simulink model "svpwm_twolevel"  (R2020a)
settings: Solver=ode45  StartTime=0.0  StopTime=0.05  RelTol=1e-3  EnableMultiTasking=on
libraries: powerlib x15, simulink x1
settings Model: Creator=Lenovo  LastModifiedBy=DELL
settings DataIOCC: LimitDataPoints=on  SaveFormat=Array  ReturnWorkspaceOutputs=off
settings OptimizationCC: LifeSpan=inf
settings DebuggingCC: SFUnexpectedBacktrackingDiag=warning  SFNoUnconditionalDefaultTransitionDiag=warning  SFExecutionAtInitializationDiag=none  ArithmeticOperatorsInVariantConditions=warning
settings HardwareCC: ProdBitPerPointer=32  ProdBitPerSizeT=32  ProdBitPerPtrDiffT=32  ProdLargestAtomicFloat=None  ProdIntDivRoundTo=Undefined  ProdEndianess=Unspecified  ProdWordSize=32  ProdHWDeviceType=32-bit Generic
settings ModelReferenceCC: PropagateSignalLabelsOutOfModel=off
settings SFSimCC: SimUseLocalCustomCode=off  CustomCodeUndefinedFunction=UseInterfaceOnly
settings RTWCC: RTWUseLocalCustomCode=off
settings CodeAppCC: StateflowObjectComments=on
settings GRTTargetCC: TargetLangStandard=C89/C90 (ANSI)
settings ConfigComp: CovMetricSettings=dw  CovHtmlReporting=on  CovSaveCumulativeToWorkspaceVar=on  CovSaveSingleToWorkspaceVar=on  CovExternalEMLEnable=off
settings SimscapeCC: SimscapeNormalizeSystem=off

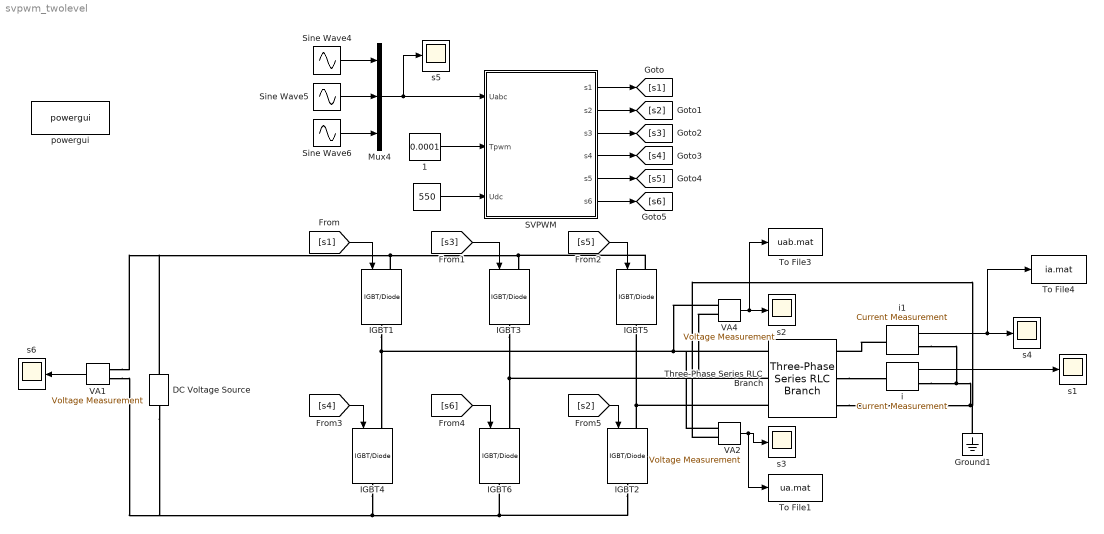
== system svpwm_twolevel ==
  " " : Constant  Value=550
  " 1" : Constant  Value=0.0001
  DC Voltage Source : powerlib/Electrical Sources/DC Voltage Source  Amplitude=550  Measurements=Voltage
  Ground1 : powerlib/Elements/Ground  LConnTagsString=a
  IGBT{1..6} (6 alike) : powerlib/Power Electronics/IGBT//Diode  Ron=1e-3  Rs=1e5  Cs=inf  Measurements=off
  Mux4 : Mux  Inputs=3
  SVPWM : Subsystem
  Sine Wave4 : Sin  Amplitude=200  Frequency=100*pi  SampleTime=0
  Sine Wave5 : Sin  Amplitude=200  Frequency=100*pi  Phase=-2*pi/3  SampleTime=0
  Sine Wave6 : Sin  Amplitude=200  Frequency=100*pi  Phase=-4*pi/3  SampleTime=0
  Three-Phase Series RLC Branch : powerlib/Elements/Three-Phase Series RLC Branch  LConnTagsString=A|B|C  RConnTagsString=A|B|C  BranchType=RL  Resistance=10  Inductance=1e-2  Capacitance=1e-6  Measurements=None
  To File1 : ToFile  Filename=ua.mat
  To File3 : ToFile  Filename=uab.mat
  To File4 : ToFile  Filename=ia.mat
  VA1 : powerlib/Measurements/Voltage Measurement  PhasorSimulation=off  OutputType=Complex  PSBequivalent=0
  VA2 : powerlib/Measurements/Voltage Measurement  PhasorSimulation=off  OutputType=Complex  PSBequivalent=0
  VA4 : powerlib/Measurements/Voltage Measurement  PhasorSimulation=off  OutputType=Complex  PSBequivalent=0
  i : powerlib/Measurements/Current Measurement  PhasorSimulation=off  OutputType=Complex  PSBequivalent=0
  i1 : powerlib/Measurements/Current Measurement  PhasorSimulation=off  OutputType=Complex  PSBequivalent=0
  powergui : powerlib/powergui  Priority=1  SimulationMode=Continuous  SampleTime=1e-6  frequency=60  Iterations=50  frequencyindice=0  Pbase=100e6  ErrMax=1e-4  UnitsV=V  UnitsW=MW  buscounter=0  FunctionMessages=off  echomessages=off  EnableUseOfTLC=off  CurrentSourceSwitches=off  DisableSnubberDevices=off  DisableRonSwitches=off  DisableVfSwitches=off  DisplayEquations=off  AutomaticDiscreteSolvers=off  SolverType=Tustin/Backward Euler (TBE)  Interpol=off  ExternalGateDelay=off  methode=off  Ts=100  x0status=blocks  SPID=off  SwTol=0  HookPort=off  NonlinearTolerance=1e-4  nMaxIteration=100  ContinueOnMaxIteration=off  RestoreLinks=warning  ResistiveCurrentMeasurement=off  Frange=[0:2:500]  Ylog=off  Xlog=on  ShowGrid=off  save=off  variable=ZData  structure=aa3  ZoomFFT=off  StartTime=0.5  cycles=19  DisplayStyle=1  fundamental=50  FreqAxis=off  MaxFrequency=770  frequencyindicesteady=1  RmsSteady=1  display=off
  s{1..6} (6 alike) : Scope
  wires:
  Mux4/1 -> s5/1, SVPWM/1(Uabc)
  " "/1 -> SVPWM/3(Udc)
  " 1"/1 -> SVPWM/2(Tpwm)
  Sine Wave4/1 -> Mux4/1
  Sine Wave5/1 -> Mux4/2
  Sine Wave6/1 -> Mux4/3
  SVPWM/1(s1) -> [s1]
  SVPWM/2(s2) -> [s2]
  SVPWM/3(s3) -> [s3]
  SVPWM/4(s4) -> [s4]
  SVPWM/5(s5) -> [s5]
  SVPWM/6(s6) -> [s6]
  [s1] -> IGBT1/1
  [s3] -> IGBT3/1
  [s5] -> IGBT5/1
  [s4] -> IGBT4/1
  [s6] -> IGBT6/1
  [s2] -> IGBT2/1
  VA1/1 -> s6/1
  i/1 -> s1/1
  VA4/1 -> To File3/1, s2/1
  VA2/1 -> To File1/1, s3/1
  i1/1 -> To File4/1, s4/1
  connections:
  IGBT1/LConn1 -- DC Voltage Source/RConn1 -- VA1/LConn1 -- IGBT5/LConn1 -- IGBT3/LConn1
  IGBT4/RConn1 -- DC Voltage Source/LConn1 -- VA1/LConn2 -- IGBT6/RConn1 -- IGBT2/RConn1
  IGBT1/RConn1 -- VA2/LConn1 -- Three-Phase Series RLC Branch/LConn1 -- VA4/LConn1 -- IGBT4/LConn1
  IGBT2/LConn1 -- IGBT5/RConn1 -- Three-Phase Series RLC Branch/LConn3
  IGBT3/RConn1 -- VA4/LConn2 -- Three-Phase Series RLC Branch/LConn2 -- IGBT6/LConn1
  Three-Phase Series RLC Branch/RConn2 -- i/LConn1
  i/RConn1 -- i1/RConn1 -- Ground1/LConn1 -- VA2/LConn2 -- Three-Phase Series RLC Branch/RConn3
  i1/LConn1 -- Three-Phase Series RLC Branch/RConn1

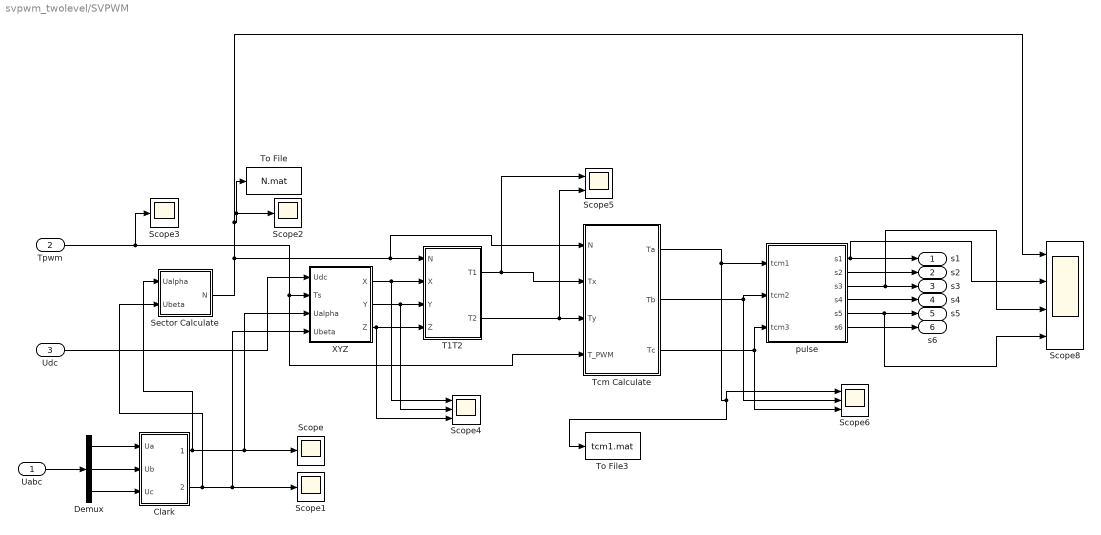
== system svpwm_twolevel/SVPWM ==
  Uabc : Inport
  Tpwm : Inport  Port=2
  Udc : Inport  Port=3
  Clark : Subsystem
  Demux : Demux  Outputs=3
  Scope{,1..3} (4 alike) : Scope
  Scope4 : Scope  NumInputPorts=3
  Scope5 : Scope  NumInputPorts=2
  Scope6 : Scope  NumInputPorts=3
  Scope8 : Scope  NumInputPorts=4
  Sector Calculate : Subsystem
  T1T2 : Subsystem
  Tcm Calculate : Subsystem
  To File : ToFile  Filename=N.mat
  To File3 : ToFile  Filename=tcm1.mat
  XYZ : Subsystem
  pulse : Subsystem
  s1 : Outport
  s2 : Outport  Port=2
  s3 : Outport  Port=3
  s4 : Outport  Port=4
  s5 : Outport  Port=5
  s6 : Outport  Port=6
  wires:
  XYZ/1(X) -> Scope4/1, T1T2/2(X)
  XYZ/2(Y) -> Scope4/2, T1T2/3(Y)
  XYZ/3(Z) -> Scope4/3, T1T2/4(Z)
  Udc/1 -> XYZ/1(Udc)
  Tpwm/1 -> Scope3/1, Tcm Calculate/4(T_PWM), XYZ/2(Ts)
  Clark/1(Ualpha) -> Sector Calculate/1(Ualpha), Scope/1, XYZ/3(Ualpha)
  Clark/2(Ubeta) -> Sector Calculate/2(Ubeta), Scope1/1, XYZ/4(Ubeta)
  Demux/3 -> Clark/3(Uc)
  Demux/2 -> Clark/2(Ub)
  Demux/1 -> Clark/1(Ua)
  Uabc/1 -> Demux/1
  T1T2/1("T1 ") -> Scope5/1, Tcm Calculate/2(Tx)
  T1T2/2(T2) -> Scope5/2, Tcm Calculate/3(Ty)
  Sector Calculate/1("N ") -> Scope8/1, To File/1, Scope2/1, Tcm Calculate/1(N), T1T2/1(N)
  Tcm Calculate/2(Tb) -> pulse/2(tcm2), Scope6/2
  Tcm Calculate/3(Tc) -> pulse/3(tcm3), Scope6/3
  Tcm Calculate/1(Ta) -> To File3/1, Scope6/1, pulse/1(tcm1)
  pulse/2(s2) -> s2/1
  pulse/3(s3) -> Scope8/3, s3/1
  pulse/4(s4) -> s4/1
  pulse/5(s5) -> Scope8/4, s5/1
  pulse/6(s6) -> s6/1
  pulse/1(s1) -> Scope8/2, s1/1

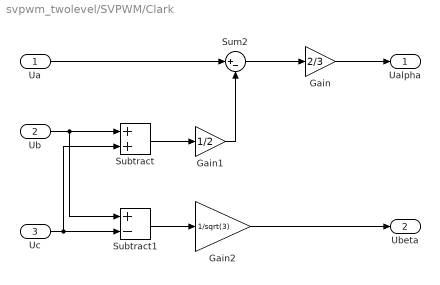
== system svpwm_twolevel/SVPWM/Clark ==
  Ua : Inport
  Ub : Inport  Port=2
  Uc : Inport  Port=3
  Gain : Gain  Gain=2/3
  Gain1 : Gain  Gain=1/2
  Gain2 : Gain  Gain=1/sqrt(3)
  Subtract : Sum
  Subtract1 : Sum  Inputs=+-
  Sum2 : Sum  Inputs=|+-
  Ualpha : Outport
  Ubeta : Outport  Port=2
  wires:
  Ua/1 -> Sum2/1
  Sum2/1 -> Gain/1
  Subtract/1 -> Gain1/1
  Gain1/1 -> Sum2/2
  Gain/1 -> Ualpha/1
  Ub/1 -> Subtract1/1, Subtract/1
  Uc/1 -> Subtract/2, Subtract1/2
  Subtract1/1 -> Gain2/1
  Gain2/1 -> Ubeta/1

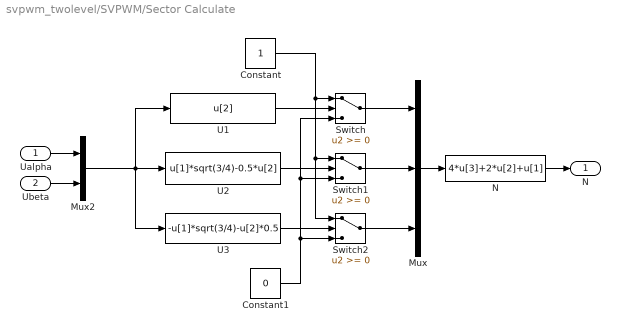
== system svpwm_twolevel/SVPWM/Sector Calculate ==
  Ualpha : Inport
  Ubeta : Inport  Port=2
  Constant : Constant
  Constant1 : Constant  Value=0
  Mux : Mux  Inputs=3
  Mux2 : Mux  Inputs=2
  N : Fcn  Expr=4*u[3]+2*u[2]+u[1]
  Switch : Switch
  Switch1 : Switch
  Switch2 : Switch
  U1 : Fcn  Expr=u[2]
  U2 : Fcn  Expr=u[1]*sqrt(3/4)-0.5*u[2]
  U3 : Fcn  Expr=-u[1]*sqrt(3/4)-u[2]*0.5
  "N " : Outport  VectorParamsAs1DForOutWhenUnconnected=off
  wires:
  Switch2/1 -> Mux/3
  Switch/1 -> Mux/1
  Ualpha/1 -> Mux2/1
  Ubeta/1 -> Mux2/2
  Mux2/1 -> U1/1, U3/1, U2/1
  U1/1 -> Switch/2
  U2/1 -> Switch1/2
  U3/1 -> Switch2/2
  Constant/1 -> Switch/1, Switch2/1, Switch1/1
  Constant1/1 -> Switch/3, Switch1/3, Switch2/3
  Switch1/1 -> Mux/2
  Mux/1 -> N/1
  N/1 -> "N "/1

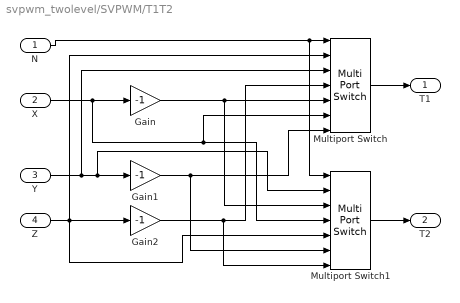
== system svpwm_twolevel/SVPWM/T1T2 ==
  N : Inport
  X : Inport  Port=2
  Y : Inport  Port=3
  Z : Inport  Port=4
  Gain : Gain  Gain=-1
  Gain1 : Gain  Gain=-1
  Gain2 : Gain  Gain=-1
  Multiport Switch : MultiPortSwitch  Inputs=6
  Multiport Switch1 : MultiPortSwitch  Inputs=6
  "T1 " : Outport
  T2 : Outport  Port=2
  wires:
  X/1 -> Multiport Switch1/4, Multiport Switch/6, Gain/1
  Y/1 -> Multiport Switch/3, Multiport Switch1/2, Gain1/1
  Z/1 -> Multiport Switch1/5, Multiport Switch/2, Gain2/1
  N/1 -> Multiport Switch1/1, Multiport Switch/1
  Gain/1 -> Multiport Switch1/3, Multiport Switch/5
  Gain2/1 -> Multiport Switch1/7, Multiport Switch/4
  Gain1/1 -> Multiport Switch1/6, Multiport Switch/7
  Multiport Switch/1 -> "T1 "/1
  Multiport Switch1/1 -> T2/1

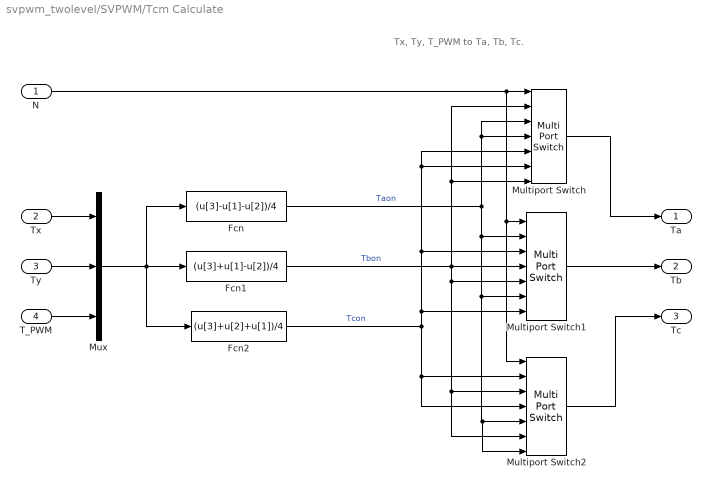
== system svpwm_twolevel/SVPWM/Tcm Calculate ==
  note: Tx, Ty, T_PWM to Ta, Tb, Tc.
  N : Inport
  Tx : Inport  Port=2
  Ty : Inport  Port=3
  T_PWM : Inport  Port=4
  Fcn : Fcn  Expr=(u[3]-u[1]-u[2])/4
  Fcn1 : Fcn  Expr=(u[3]+u[1]-u[2])/4
  Fcn2 : Fcn  Expr=(u[3]+u[2]+u[1])/4
  Multiport Switch : MultiPortSwitch  Inputs=6
  Multiport Switch1 : MultiPortSwitch  Inputs=6
  Multiport Switch2 : MultiPortSwitch  Inputs=6
  Mux : Mux  Inputs=3
  Ta : Outport
  Tb : Outport  Port=2
  Tc : Outport  Port=3
  wires:
  Mux/1 -> Fcn2/1, Fcn/1, Fcn1/1
  T_PWM/1 -> Mux/3
  Ty/1 -> Mux/2
  Tx/1 -> Mux/1
  Multiport Switch2/1 -> Tc/1
  Multiport Switch1/1 -> Tb/1
  Multiport Switch/1 -> Ta/1
  Fcn/1 -> Multiport Switch/3, Multiport Switch/4, Multiport Switch1/6, Multiport Switch2/5, Multiport Switch2/7, Multiport Switch1/2  "Taon"
  Fcn1/1 -> Multiport Switch1/5, Multiport Switch2/3, Multiport Switch2/6, Multiport Switch1/4, Multiport Switch/7, Multiport Switch/2  "Tbon"
  Fcn2/1 -> Multiport Switch/5, Multiport Switch/6, Multiport Switch1/3, Multiport Switch1/7, Multiport Switch2/2, Multiport Switch2/4  "Tcon"
  N/1 -> Multiport Switch2/1, Multiport Switch1/1, Multiport Switch/1

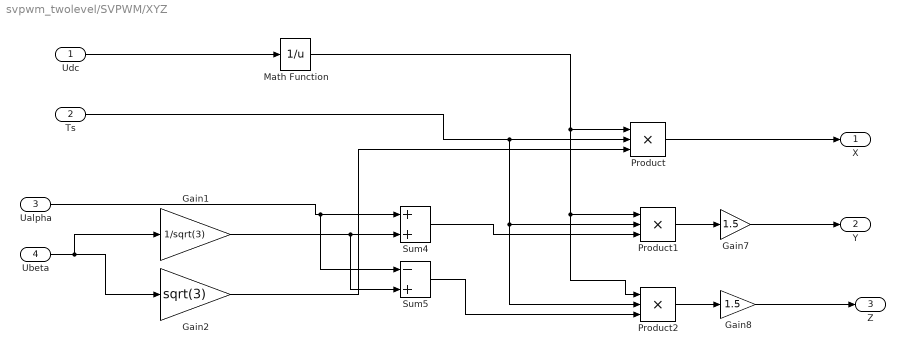
== system svpwm_twolevel/SVPWM/XYZ ==
  Udc : Inport
  Ts : Inport  Port=2
  Ualpha : Inport  Port=3
  Ubeta : Inport  Port=4
  Gain1 : Gain  Gain=1/sqrt(3)  SaturateOnIntegerOverflow=on  OutDataTypeStr=Inherit: Same as input  ParamDataTypeStr=Inherit: Same as input
  Gain2 : Gain  Gain=sqrt(3)  SaturateOnIntegerOverflow=on  OutDataTypeStr=Inherit: Same as input  ParamDataTypeStr=Inherit: Same as input
  Gain7 : Gain  Gain=1.5  SaturateOnIntegerOverflow=on  OutDataTypeStr=Inherit: Same as input  ParamDataTypeStr=Inherit: Same as input
  Gain8 : Gain  Gain=1.5  SaturateOnIntegerOverflow=on  OutDataTypeStr=Inherit: Same as input  ParamDataTypeStr=Inherit: Same as input
  Math Function : Math  Operator=reciprocal  SignedPower=on  SaturateOnIntegerOverflow=on
  Product : Product  Inputs=3
  Product1 : Product  Inputs=3
  Product2 : Product  Inputs=3
  Sum4 : Sum  InputSameDT=on  SaturateOnIntegerOverflow=on  OutDataTypeStr=Inherit: Same as first input
  Sum5 : Sum  Inputs=-+  InputSameDT=on  SaturateOnIntegerOverflow=on  OutDataTypeStr=Inherit: Same as first input
  X : Outport
  Y : Outport  Port=2
  Z : Outport  Port=3
  wires:
  Sum4/1 -> Product1/3
  Sum5/1 -> Product2/3
  Product/1 -> X/1
  Product2/1 -> Gain8/1
  Product1/1 -> Gain7/1
  Math Function/1 -> Product/1, Product2/1, Product1/1
  Gain8/1 -> Z/1
  Gain7/1 -> Y/1
  Udc/1 -> Math Function/1
  Ts/1 -> Product2/2, Product1/2, Product/2
  Ualpha/1 -> Sum5/1, Sum4/1
  Gain1/1 -> Sum5/2, Sum4/2
  Gain2/1 -> Product/3
  Ubeta/1 -> Gain1/1, Gain2/1

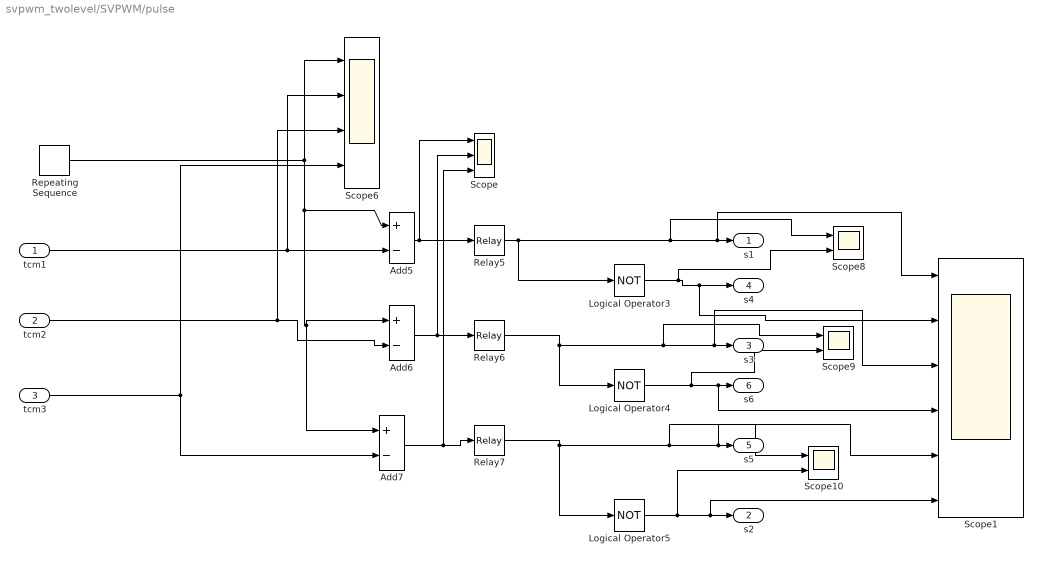
== system svpwm_twolevel/SVPWM/pulse ==
  tcm1 : Inport
  tcm2 : Inport  Port=2
  tcm3 : Inport  Port=3
  Add5 : Sum  Inputs=+-
  Add6 : Sum  Inputs=+-
  Add7 : Sum  Inputs=+-
  Logical Operator3 : Logic  Operator=NOT  AllPortsSameDT=off  OutDataTypeStr=boolean
  Logical Operator4 : Logic  Operator=NOT  AllPortsSameDT=off  OutDataTypeStr=boolean
  Logical Operator5 : Logic  Operator=NOT  AllPortsSameDT=off  OutDataTypeStr=boolean
  Relay5 : Relay
  Relay6 : Relay
  Relay7 : Relay
  Repeating Sequence : simulink/Sources/Repeating Sequence  rep_seq_t=[0 0.00005 0.0001]  rep_seq_y=[0 0.00005 0]
  Scope : Scope  NumInputPorts=3
  Scope1 : Scope  NumInputPorts=6
  Scope10 : Scope  NumInputPorts=2
  Scope6 : Scope  NumInputPorts=4
  Scope8 : Scope  NumInputPorts=2
  Scope9 : Scope  NumInputPorts=2
  s1 : Outport
  s2 : Outport  Port=2
  s3 : Outport  Port=3
  s4 : Outport  Port=4
  s5 : Outport  Port=5
  s6 : Outport  Port=6
  wires:
  tcm2/1 -> Scope6/3, Add6/2
  Add6/1 -> Scope/2, Relay6/1
  Add7/1 -> Scope/3, Relay7/1
  Relay7/1 -> Scope1/5, s5/1, Scope10/1, Logical Operator5/1
  tcm1/1 -> Scope6/2, Add5/2
  Repeating Sequence/1 -> Add5/1, Add7/1, Add6/1, Scope6/1
  tcm3/1 -> Add7/2, Scope6/4
  Relay5/1 -> Logical Operator3/1, Scope1/1, s1/1, Scope8/1
  Logical Operator3/1 -> Scope1/2, s4/1, Scope8/2
  Logical Operator5/1 -> Scope1/6, s2/1, Scope10/2
  Logical Operator4/1 -> Scope1/4, s6/1, Scope9/2
  Relay6/1 -> Scope1/3, s3/1, Scope9/1, Logical Operator4/1
  Add5/1 -> Scope/1, Relay5/1
